simulink model "ASS3_Trial1"  (R2023a)
settings: Solver=FixedStepAuto  StartTime=0.0  StopTime=100  RelTol=1e-3
undefined symbols (not defined in the file): DiscIntNeverNeededParam
libraries: dspadpt3 x4, dspstat3 x4, dspsrcs4 x1, fuzblock x1
settings Model: Creator=Asus  LastModifiedBy=Aditya Prachand
settings OptimizationCC: EnhancedBackFolding=on  PassReuseOutputArgsAs=Individual arguments  ZeroExternalMemoryAtStartup=off  ZeroInternalMemoryAtStartup=off  MaxStackSize=64  OptimizeBlockOrder=speed  DifferentSizesBufferReuse=on  OptimizationCustomize=off  EfficientTunableParamExpr=on
settings DebuggingCC: ParameterTunabilityLossMsg=error
settings HardwareCC: ProdBitPerLong=64  ProdLargestAtomicInteger=LongLong  ProdLargestAtomicFloat=Double  ProdLongLongMode=on  ProdHWDeviceType=ARM Compatible->ARM 64-bit (LP64)
settings SFSimCC: MATLABDynamicMemAlloc=off
settings RTWCC: Description=Embedded Coder  SystemTargetFile=ert.tlc  HardwareBoard=Android Device (64bit)  TLCOptions="-aInlineSetEventsForThisBaseRateFcn=TLC_FALSE -aSuppressMultiTaskScheduler=TLC_FALSE  -aRateBasedStepFcn=0"  TemplateMakefile=ert_default_tmf  RTWVerbose=off  Toolchain=Android SDK/NDK Tools
settings CodeAppCC: ForceParamTrailComments=on  IgnoreCustomStorageClasses=off  OperatorAnnotations=on  SimulinkDataObjDesc=on  SFDataObjDesc=on  InsertBlockDesc=on

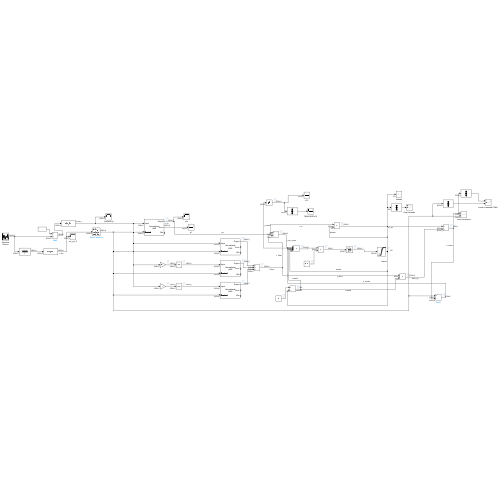
[thumbnail: Simulink's stored preview of the top-level diagram]
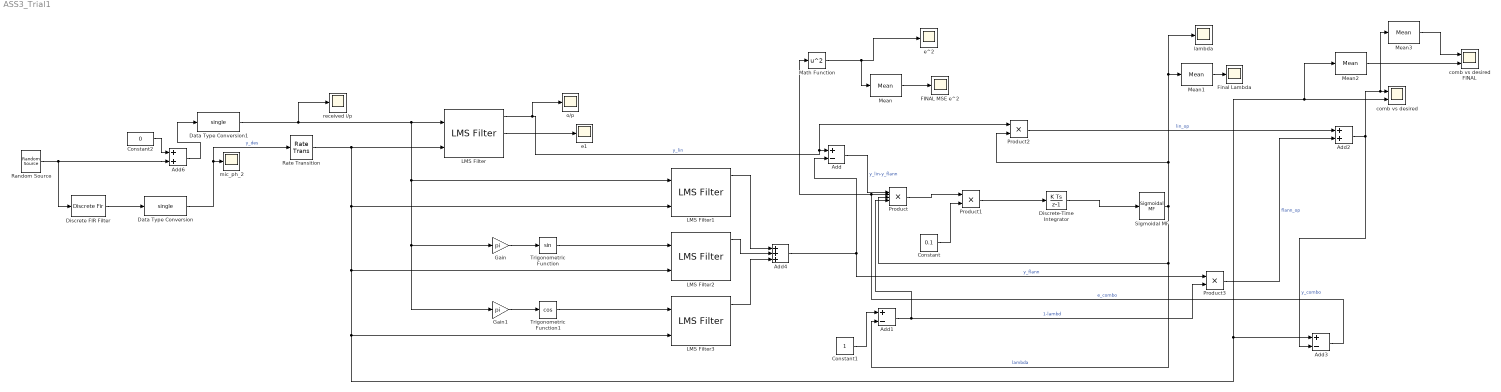
== system ASS3_Trial1 ==
  Add : Sum  Inputs=+-
  Add1 : Sum  Inputs=+-
  Add2 : Sum
  Add3 : Sum  Inputs=+-
  Add4 : Sum  Inputs=+++
  Add6 : Sum
  Constant : Constant  Value=0.1
  Constant1 : Constant
  Constant2 : Constant  Value=0  OutDataTypeStr=single
  Data Type Conversion : DataTypeConversion  OutDataTypeStr=single  SaturateOnIntegerOverflow=off  RndMeth=Floor
  Data Type Conversion1 : DataTypeConversion  OutDataTypeStr=single  SaturateOnIntegerOverflow=off  RndMeth=Floor
  Discrete FIR Filter : DiscreteFir  Coefficients=[1, 0.5, -0.2, 0.1, -0.05]  InputProcessing=Columns as channels (frame based)
  Discrete-Time Integrator : DiscreteIntegrator  SampleTime=-1  ICPrevOutput=DiscIntNeverNeededParam  ICPrevScaledInput=DiscIntNeverNeededParam
  FINAL MSE e^2 : Scope
  Final Lambda : Scope
  Gain : Gain  Gain=pi
  Gain1 : Gain  Gain=pi
  LMS Filter : dspadpt3/LMS Filter  Algo=Normalized LMS  L=4  stepflag=Dialog  mu=0.1  leakage=1.0  ic=0  Adapt=off  resetflag=None  weights=on  addnparflag=off  roundingMode=Floor  overflowMode=on  firstCoeffMode=Specify word length  firstCoeffWordLength=16  firstCoeffFracLength=15
  LMS Filter1 : dspadpt3/LMS Filter  Algo=Normalized LMS  L=96  stepflag=Dialog  mu=0.001  leakage=1.0  ic=0  Adapt=off  resetflag=None  weights=on  addnparflag=off  roundingMode=Floor  overflowMode=off
  LMS Filter2 : dspadpt3/LMS Filter  Algo=Normalized LMS  L=96  stepflag=Dialog  mu=0.001  leakage=1.0  ic=0  Adapt=off  resetflag=None  weights=on  addnparflag=off  roundingMode=Floor  overflowMode=off
  LMS Filter3 : dspadpt3/LMS Filter  Algo=Normalized LMS  L=96  stepflag=Dialog  mu=0.001  leakage=1.0  ic=0  Adapt=off  resetflag=None  weights=on  addnparflag=off  roundingMode=Floor  overflowMode=off
  Math Function : Math  Operator=square
  Mean{,1..3} (4 alike) : dspstat3/Mean  run=off  InputProcessing=Columns as channels (frame based)  reset_popup=None  directionMode=Entire input  dimension=1  roiEnable=off  roiType=Rectangles  roiPortion=Entire ROI  roiOutput=Individual statistics for each ROI  roiFlag=off  roundingMode=Floor  overflowMode=off  outputDataTypeStr=Inherit: Same as accumulator  outputMin=[]  outputMax=[]  outputLastDataTypeStr=Inherit: Same as accumulator
  Product : Product  Inputs=4
  Product1 : Product
  Product2 : Product
  Product3 : Product
  Random Source : dspsrcs4/Random Source  SrcType=Gaussian  NormMethod=Ziggurat  CltLength=12  MinVal=0  MaxVal=1  MeanVal=0  VarVal=1  RepMode=Not repeatable  rawSeed=1  IsInherit=off  SampMode=Discrete  SampTime=1/16000  SampFrame=255  DataType=Single  OutComplex=Real  OutputFrames=off
  Rate Transition : RateTransition  Integrity=off  OutPortSampleTimeOpt=Inherit
  Sigmoidal MF : fuzblock/Membership  Functions/Sigmoidal MF  a=1  c=0
  Trigonometric Function : Trigonometry
  Trigonometric Function1 : Trigonometry  Operator=cos
  comb vs desired : Scope  NumInputPorts=2
  comb vs desired FINAL : Scope  NumInputPorts=2
  e1 : Scope
  e^2 : Scope
  lambda : Scope
  mic_ph_2 : Scope
  o/p : Scope
  received i/p : Scope
  wires:
  Gain1/1 -> Trigonometric Function1/1
  Gain/1 -> Trigonometric Function/1
  Trigonometric Function/1 -> LMS Filter2/1
  Trigonometric Function1/1 -> LMS Filter3/1
  LMS Filter/1 -> Product2/1, Add/1, o/p/1  "y_lin"
  Add/1 -> Product/1  "y_lin-y_flann"
  Constant1/1 -> Add1/1
  Product/1 -> Product1/1
  Constant/1 -> Product1/2
  Product1/1 -> Discrete-Time Integrator/1
  Discrete-Time Integrator/1 -> Sigmoidal MF/1
  Sigmoidal MF/1 -> Mean1/1, lambda/1, Product2/2, Add1/2, Product/3  "lambda"
  Add1/1 -> Product/4, Product3/2  "1-lambd"
  Product2/1 -> Add2/1  "lin_op"
  Product3/1 -> Add2/2  "flann_op"
  Add2/1 -> Mean3/1, comb vs desired/1, Add3/2  "y_combo"
  Add3/1 -> Math Function/1, Product/2  "e_combo"
  Data Type Conversion/1 -> mic_ph_2/1, Rate Transition/1  "y_des"
  Add4/1 -> Add/2, Product3/1  "y_flann"
  LMS Filter1/1 -> Add4/1
  LMS Filter2/1 -> Add4/2
  LMS Filter3/1 -> Add4/3
  LMS Filter/2 -> e1/1
  Random Source/1 -> Add6/2, Discrete FIR Filter/1
  Data Type Conversion1/1 -> LMS Filter/1, LMS Filter1/1, Gain1/1, Gain/1, received i/p/1
  Constant2/1 -> Add6/1
  Add6/1 -> Data Type Conversion1/1
  Math Function/1 -> Mean/1, e^2/1
  Rate Transition/1 -> LMS Filter/2, Add3/1, Mean2/1, comb vs desired/2, LMS Filter3/2, LMS Filter2/2, LMS Filter1/2
  Mean/1 -> FINAL MSE e^2/1
  Mean1/1 -> Final Lambda/1
  Mean2/1 -> comb vs desired FINAL/2
  Mean3/1 -> comb vs desired FINAL/1
  Discrete FIR Filter/1 -> Data Type Conversion/1
